simulink model "vipsurveillance"  (R2015b)
settings: Solver=FixedStepDiscrete  SolverMode=SingleTasking  StartTime=0.0  StopTime=inf  RelTol=1e-3
undefined symbols (not defined in the file or in its folder): gray
libraries: visionsinks x2, visiontextngfix x1, vipmisc x1, visionanalysis x1, dspvision x1
settings Model: FPTRunName=Active  ExtModeAutoUpdateStatusClock=off  Creator=The MathWorks, Inc.  LastModifiedBy=The MathWorks, Inc.
settings DataIOCC: SaveFormat=Array  SaveOutput=off  SaveTime=off  SignalLoggingName=sigsOut
settings OptimizationCC: ExpressionDepthLimit=2147483647  InitFltsAndDblsToZero=on  EfficientMapNaN2IntZero=off
settings DebuggingCC: SaveWithParameterizedLinksMsg=none  CheckExecutionContextPreStartOutputMsg=on  CheckExecutionContextRuntimeOutputMsg=on  SignalResolutionControl=TryResolveAllWithWarning  MultiTaskDSMMsg=warning  MultiTaskCondExecSysMsg=none  ParameterPrecisionLossMsg=none  FcnCallInpInsideContextMsg=UseLocalSettings  StateNameClashWarn=warning  StrictBusMsg=None
settings HardwareCC: ProdBitPerPointer=32  ProdLargestAtomicFloat=None  ProdIntDivRoundTo=Undefined  ProdEndianess=Unspecified  ProdWordSize=32  ProdHWDeviceType=32-bit Generic  TargetBitPerLong=64  TargetBitPerPointer=64  TargetLongLongMode=on  TargetIntDivRoundTo=Zero  TargetEndianess=LittleEndian  TargetWordSize=64  TargetHWDeviceType=Generic->MATLAB Host Computer  ProdEqTarget=off
settings GRTTargetCC: TargetFcnLib=ansi_tfl_tmw.mat  GeneratePreprocessorConditionals=Disable all  CombineOutputUpdateFcns=off  GRTInterface=on
settings ConfigComp: CovModelRefEnable=Off  CovSFcnEnable=off

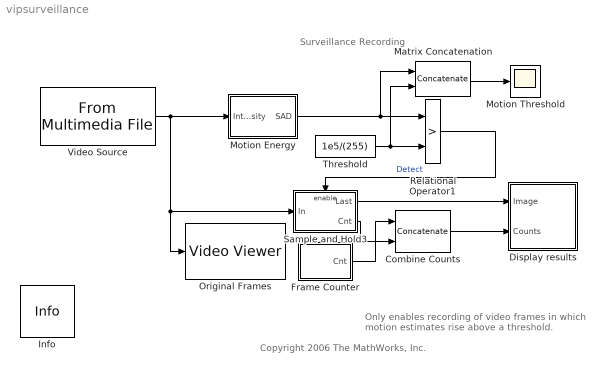
== system vipsurveillance ==
  note: Only enables recording of video frames in
      | which motion estimates rise above a threshold.
  note: Surveillance Recording
  note: Copyright 2006 The MathWorks, Inc.
  Combine Counts : Concatenate  Mode=Multidimensional array  ConcatenateDimension=2
  Display results : Subsystem
  Frame Counter : Subsystem
  Info : vipmisc/Info  SystemSampleTime=-1
  Matrix Concatenation : Concatenate  Mode=Multidimensional array  ConcatenateDimension=2
  Motion Threshold : Scope
  Motion Energy : Subsystem
  Original Frames : visionsinks/Video Viewer  inputType=Obsolete7b  imagePorts=One multidimensional signal  useColorMap=off  colormapValue=gray(256)  specRange=off  minInputVal=0  maxInputVal=255  FigPos=[66 266 166 165]  AxisZoom=on  trueSizedOnce=on  OpenAtMdlStart=on  DefaultConfigurationName=vipscopes.VideoViewerScopeCfg
  Relational Operator1 : RelationalOperator  Operator=>  OutDataTypeStr=boolean  InputSameDT=on
  Sample and Hold3 : Subsystem  TreatAsAtomicUnit=on
  Threshold : Constant  Value=1e5/(255)  VectorParams1D=off  OutDataTypeStr=Inherit: Inherit via back propagation
  Video Source : dspvision/From Multimedia File  inputFilename=vipmen.avi  loop=on  numPlays=inf  outputStreams=Video only  videoDataType=single  audioDataType=int16  inheritSampleTime=on  userDefinedSampleTime=1/30  noAudioOutput=off  isIntensityVideo=off  fourcc=Intensity  colorVideoFormat=Separate color signals  outputEOF=off  dataOrg=Column-major  audioFrameSize=1024  computeAudioFrameSize=off  outSamplingMode=Frame based
  wires:
  Motion Energy/1(SAD) -> Matrix Concatenation/1, Relational Operator1/1
  Threshold/1 -> Matrix Concatenation/2, Relational Operator1/2
  Relational Operator1/1 -> Sample and Hold3/Enable  "Detect"
  Sample and Hold3/2(" Cnt") -> Combine Counts/2
  Combine Counts/1 -> Display results/2(Counts)
  Matrix Concatenation/1 -> Motion Threshold/1
  Frame Counter/1(" Cnt") -> Combine Counts/1
  Video Source/1 -> Sample and Hold3/1(In), Original Frames/1, Motion Energy/1(Intensity)
  Sample and Hold3/1(Last) -> Display results/1(Image)

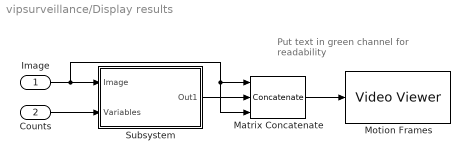
== system vipsurveillance/Display results ==
  note: Put text in green
      | channel for readability
  Image : Inport
  Counts : Inport  Port=2
  Matrix Concatenate : Concatenate  NumInputs=3  Mode=Multidimensional array  ConcatenateDimension=3
  Motion Frames : visionsinks/Video Viewer  inputType=Obsolete7b  imagePorts=One multidimensional signal  useColorMap=off  colormapValue=gray(256)  specRange=off  minInputVal=0  maxInputVal=255  FigPos=[253 260 167 159]  AxisZoom=on  trueSizedOnce=on  OpenAtMdlStart=on  DefaultConfigurationName=vipscopes.VideoViewerScopeCfg
  Subsystem : Subsystem
  wires:
  Counts/1 -> Subsystem/2(Variables)
  Matrix Concatenate/1 -> Motion Frames/1
  Subsystem/1(Out1) -> Matrix Concatenate/2
  Image/1 -> Subsystem/1(Image), Matrix Concatenate/1, Matrix Concatenate/3

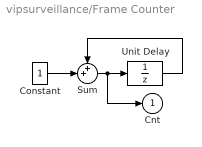
== system vipsurveillance/Frame Counter ==
  Constant : Constant  OutDataTypeStr=int32
  Sum : Sum  Inputs=++|  OutDataTypeStr=Inherit: Same as first input
  Unit Delay : UnitDelay  SampleTime=-1
  " Cnt" : Outport
  wires:
  Constant/1 -> Sum/2
  Sum/1 -> " Cnt"/1, Unit Delay/1
  Unit Delay/1 -> Sum/1

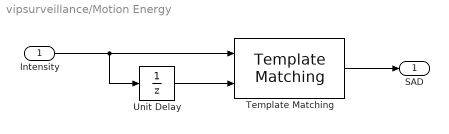
== system vipsurveillance/Motion Energy ==
  Intensity : Inport
  Template Matching : visionanalysis/Template Matching  metric=Sum of absolute differences  output=Metric matrix  method=Exhaustive  nMetric=off  nSize=3  roi=off  roiValid=off  accumMode=Binary point scaling  accumWordLength=32  accumFracLength=0  prodOutputMode=Binary point scaling  prodOutputWordLength=32  prodOutputFracLength=0  roundingMode=Floor  overflowMode=off
  Unit Delay : UnitDelay  SampleTime=-1
  SAD : Outport
  wires:
  Template Matching/1 -> SAD/1
  Unit Delay/1 -> Template Matching/2
  Intensity/1 -> Template Matching/1, Unit Delay/1

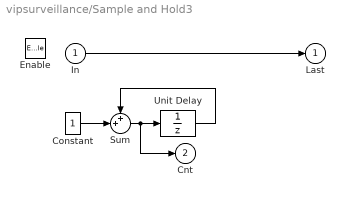
== system vipsurveillance/Sample and Hold3 ==
  In : Inport
  Enable : EnablePort  PropagateVarSize=During execution
  Constant : Constant  OutDataTypeStr=int32
  Sum : Sum  Inputs=++|  OutDataTypeStr=Inherit: Same as first input
  Unit Delay : UnitDelay  SampleTime=-1
  Last : Outport
  " Cnt" : Outport  Port=2
  wires:
  Unit Delay/1 -> Sum/1
  Sum/1 -> " Cnt"/1, Unit Delay/1
  Constant/1 -> Sum/2
  In/1 -> Last/1

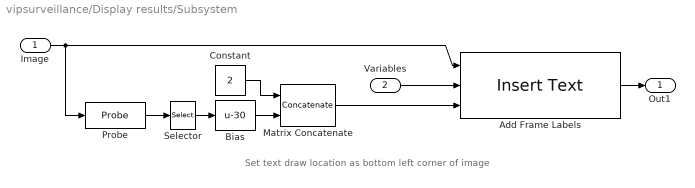
== system vipsurveillance/Display results/Subsystem ==
  note: Set text draw location as bottom left corner of image
  Image : Inport
  Variables : Inport  Port=2
  Add Frame Labels : visiontextngfix/Insert Text  inputType=Obsolete  theText=['Source frame: %d' sprintf('\n') 'Captured frame: %d']  getTextLocFrom=Input port  textLoc=[90 2]  getTextColorFrom=Specify via dialog  textColor=1  getTextIntensityFrom=Specify via dialog  textIntensity=1  getTextOpacityFrom=Specify via dialog  textOpacity=1.0  dummyVar2=0  dummyVar3=0  dummyVar4=0  imagePorts=One multidimensional signal  isInputTransposed=off  fontFace=LucidaTypewriterRegular  dummyVar1=0  blockFontSize=12  antiAliased=on
  Bias : Bias  Bias=-30
  Constant : Constant  Value=2  OutDataTypeStr=int32
  Matrix Concatenate : Concatenate  Mode=Multidimensional array  ConcatenateDimension=2
  Probe : Probe  ProbeWidth=off  ProbeSampleTime=off  ProbeComplexSignal=off  ProbeSignalDimensions=on  ProbeDimensionsDataType=int32
  Selector : Selector  InputPortWidth=2  IndexOptions=Index vector (dialog)  Indices=1  OutputSizes=1
  Out1 : Outport
  wires:
  Matrix Concatenate/1 -> Add Frame Labels/3
  Selector/1 -> Bias/1
  Probe/1 -> Selector/1
  Add Frame Labels/1 -> Out1/1
  Variables/1 -> Add Frame Labels/2
  Image/1 -> Probe/1, Add Frame Labels/1
  Bias/1 -> Matrix Concatenate/2
  Constant/1 -> Matrix Concatenate/1
